simulink model "MPSK_frame_based"  (R2017b)
settings: Solver=FixedStepAuto  StartTime=0.0  StopTime=1  FixedStep=1/sampleRate  RelTol=1e-3
values from neighbouring files (symbols this model uses):
  detectionThreshold = 0.5    [MPSK_frame_based_init.m]    (also in MPSK_sample_based_init.m)
  M = 2^K    (= 4)    [Digital_QAM.m]    (also in MPSK_constellation_decisionRegions.m = 8; MPSK_frame_based_init.m = 2; MPSK_init.m = 2; MPSK_sample_based_init.m = 2)
  phaseOffset = pi    (= 3.14159265359)    [MPSK_frame_based_init.m]    (also in MPSK_init.m = -0.785398163397; MPSK_sample_based_init.m)
  sampleRate = 100    [MPSK_frame_based_init.m]    (also in MPSK_sample_based_init.m)
undefined symbols (not defined in the file or in its folder): i
libraries: simulink_extras x3, commutil2 x3, simulink x2, commfilt2 x2, commchan3 x1, dspsigops x1, commseqgen3 x1, commsink2 x1, commrflib2 x1, commrandsrc3 x1
settings Model: Creator=john3  LastModifiedBy=croft

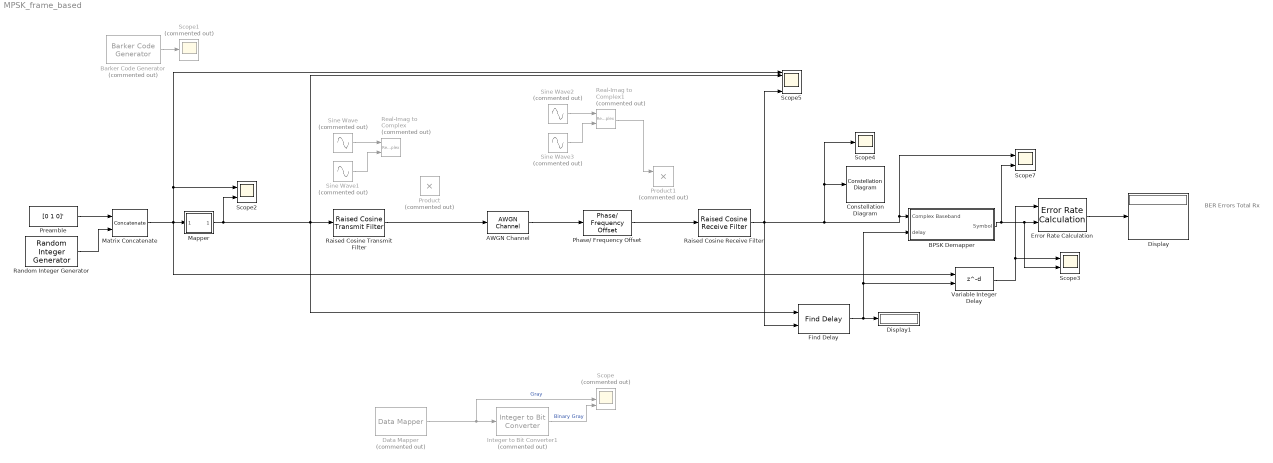
== system MPSK_frame_based ==
  note: BER
      | Errors
      | Total Rx
  AWGN Channel : commchan3/AWGN Channel  InputProcessing=Columns as channels (frame based)  seed=67  noiseMode="Signal to noise ratio  (SNR)"  EbNodB=10  EsNodB=10  SNRdB=30  bitsPerSym=K  Ps=1  Tsym=1  variance=1
  BPSK Demapper : Subsystem
  Barker Code Generator : commseqgen3/Barker Code Generator  Commented=on  Length=7  LengthSimulink=7  SampleTime=1  SamplesPerFrame=1  OutputDataType=double  SimulateUsing=Interpreted execution
      settings: SourceProductName=Communications System Toolbox  SourceProductBaseCode=CM
  Constellation Diagram : ConstellationDiagram
  Data Mapper : commutil2/Data Mapper  Commented=on  MapMode=Binary to Gray  M=M  MapVec=[0 1 3 2 7 6 4 5]
      settings: SourceProductName=Communications System Toolbox  SourceProductBaseCode=CM
  Display : Display
  Display1 : Display
  Error Rate Calculation : commsink2/Error Rate Calculation  N=0  st_delay=0  cp_mode=Entire frame  subframe=[]  PMode=Port  WsName=ErrorVec  RsMode2=off  stop=off  numErr=100  maxBits=1e6
  Find Delay : commutil2/Find Delay  corrLength=100  chgSigOP=off  stopUpdate=off  numConstDelay=3
      settings: SourceProductName=Communications System Toolbox  SourceProductBaseCode=CM
  Integer to Bit Converter1 : commutil2/Integer to Bit Converter  Commented=on  nbits=K  signedInputValues=Unsigned  bitOrder=MSB first  outDtype=Inherit via internal rule
  Mapper : Subsystem
  Matrix Concatenate : Concatenate  Mode=Multidimensional array
  Phase/ Frequency Offset : commrflib2/Phase// Frequency Offset  phaseOffset=phaseOffset*180/pi  freqPort=off  freqOffset=0
      settings: SourceProductName=Communications System Toolbox
  Preamble : Constant  Value=[0 1 0]'  SampleTime=1
  Product : Product  Commented=on
  Product1 : Product  Commented=on
  Raised Cosine Receive Filter : commfilt2/Raised Cosine Receive Filter  filtType=Square root  R=1  filtSpan=4  N=10  downFactor=10  downOffset=0  filterGain=1  InputProcessing=Columns as channels (frame based)  RateOptions=Enforce single-rate processing  framing=Mute  checkCoeff=off  variableName=rcRxFilt  currentFiltSpan=4  D=(4)/2  inputOffset=0  sampMode=Mute  saveAsFlag=0  rateMode=Downsampling  checkGain=Normalized  launchFVT=on  roundingMode=Floor  overflowMode=off  coeffDataTypeStr=Inherit: Same word length as input  coeffMin=[]  coeffMax=[]  coeffLastDataTypeStr=Inherit: Same word length as input  accumDataTypeStr=Inherit: Same as product output  accumLastDataTypeStr=Inherit: Same as product output  outputDataTypeStr=Inherit: Same as accumulator  outputMin=[]  outputMax=[]  outputLastDataTypeStr=Inherit: Same as accumulator
  Raised Cosine Transmit Filter : commfilt2/Raised Cosine Transmit Filter  filtType=Square root  R=1  filtSpan=4  N=10  filterGain=1  InputProcessing=Columns as channels (frame based)  RateOptions=Enforce single-rate processing  framing=Mute  checkCoeff=off  variableName=rcTxFilt  checkGain=Normalized  sampMode=Mute  saveAsFlag=0  currentFiltSpan=4  D=(4)/2  launchFVT=on  roundingMode=Floor  overflowMode=off  coeffDataTypeStr=Inherit: Same word length as input  coeffMin=[]  coeffMax=[]  coeffLastDataTypeStr=Inherit: Same word length as input  outputDataTypeStr=Inherit: Same as accumulator  outputMin=[]  outputMax=[]  outputLastDataTypeStr=Inherit: Same as accumulator
  Random Integer Generator : commrandsrc3/Random Integer Generator  SetSize=M  SeedSource=Auto  Seed=0  SampleTime=sampleRate  SamplesPerFrame=97  OutputDataType=double  SimulateUsing=Interpreted execution
  Real-Imag to Complex : RealImagToComplex  Commented=on
  Real-Imag to Complex1 : RealImagToComplex  Commented=on
  Scope : Scope  Commented=on  NumInputPorts=3
  Scope1 : Scope  Commented=on
  Scope2 : Scope  NumInputPorts=2
  Scope3 : Scope  NumInputPorts=2
  Scope4 : Scope
  Scope5 : Scope  NumInputPorts=7
  Scope7 : Scope  NumInputPorts=2
  Sine Wave : Sin  Commented=on  Phase=pi/2  SampleTime=0
  Sine Wave1 : Sin  Commented=on  SampleTime=0
  Sine Wave2 : Sin  Commented=on  Phase=pi/2  SampleTime=0
  Sine Wave3 : Sin  Commented=on  SampleTime=0
  Variable Integer Delay : Delay  DelayLengthSource=Input port  InputProcessing=Columns as channels (frame based)
      settings: InputPortMap=u0,p1
  wires:
  Data Mapper/1 -> Scope/2, Integer to Bit Converter1/1  "Gray"
  Integer to Bit Converter1/1 -> Scope/3  "Binary Gray"
  Raised Cosine Receive Filter/1 -> Scope5/7, Find Delay/2, Scope4/1, Constellation Diagram/1, Scope7/1, BPSK Demapper/1(Complex Baseband)
  BPSK Demapper/1(Symbol) -> Scope7/2, Scope3/2, Error Rate Calculation/2
  Error Rate Calculation/1 -> Display/1
  Barker Code Generator/1 -> Scope1/1
  Preamble/1 -> Matrix Concatenate/1
  Random Integer Generator/1 -> Matrix Concatenate/2
  Matrix Concatenate/1 -> Variable Integer Delay/1, Scope5/1, Scope2/1, Mapper/1(In1)
  Mapper/1(Out1) -> Scope5/2, Find Delay/1, Raised Cosine Transmit Filter/1, Scope2/2
  Find Delay/1 -> BPSK Demapper/2(delay), Variable Integer Delay/2, Display1/1
  Variable Integer Delay/1 -> Scope3/1, Error Rate Calculation/1
  AWGN Channel/1 -> Phase/ Frequency Offset/1
  Sine Wave/1 -> Real-Imag to Complex/1
  Sine Wave1/1 -> Real-Imag to Complex/2
  Raised Cosine Transmit Filter/1 -> AWGN Channel/1
  Sine Wave3/1 -> Real-Imag to Complex1/2
  Sine Wave2/1 -> Real-Imag to Complex1/1
  Phase/ Frequency Offset/1 -> Raised Cosine Receive Filter/1
  Real-Imag to Complex1/1 -> Product1/1

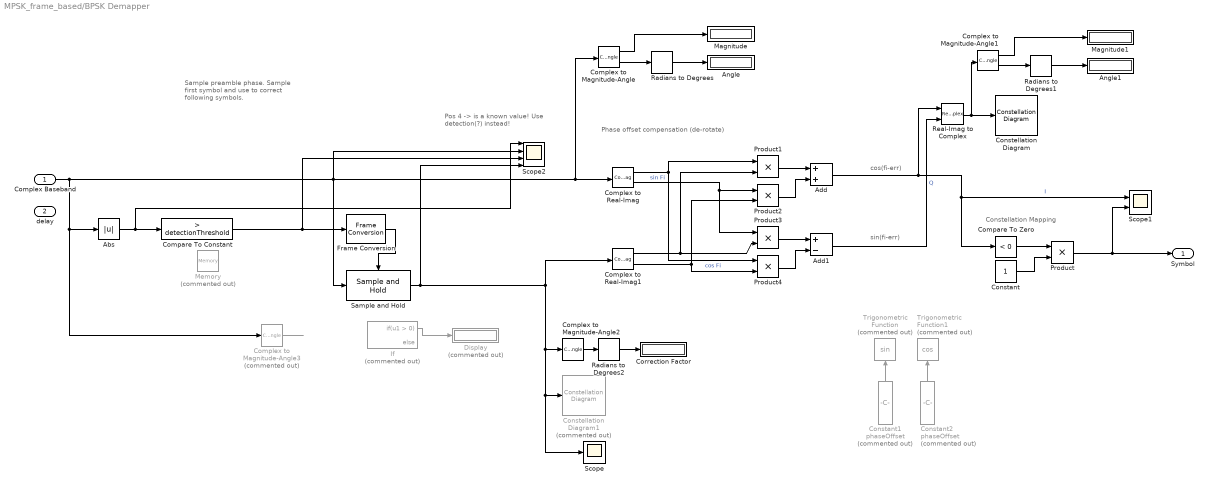
== system MPSK_frame_based/BPSK Demapper ==
  note: Pos 4 ->
      | is a known value!
      | Use detection(?)
      | instead!
  note: cos(fi-err)
  note: Sample preamble phase.
      | Sample first symbol and
      | use to correct following
      | symbols.
  note: Phase offset compensation (de-rotate)
  note: Constellation Mapping
  note: sin(fi-err)
  Complex Baseband : Inport
  delay : Inport  Port=2
  Abs : Abs
  Add : Sum
  Add1 : Sum  Inputs=+-
  Angle : Display
  Angle1 : Display
  Compare To Constant : simulink/Logic and Bit Operations/Compare To Constant  relop=>  const=detectionThreshold  OutDataTypeStr=boolean
  Compare To Zero : simulink/Logic and Bit Operations/Compare To Zero  relop=<  OutDataTypeStr=boolean
  Complex to Magnitude-Angle : ComplexToMagnitudeAngle
  Complex to Magnitude-Angle1 : ComplexToMagnitudeAngle
  Complex to Magnitude-Angle2 : ComplexToMagnitudeAngle  Output=Angle
  Complex to Magnitude-Angle3 : ComplexToMagnitudeAngle  Commented=on  Output=Angle
  Complex to Real-Imag : ComplexToRealImag
  Complex to Real-Imag1 : ComplexToRealImag
  Constant : Constant
  Constant1 : Constant  Commented=on  Value=phaseOffset
  Constant2 : Constant  Commented=on  Value=phaseOffset
  Constellation Diagram : ConstellationDiagram
  Constellation Diagram1 : ConstellationDiagram  Commented=on
  Correction Factor : Display
  Display : Display  Commented=on
  Frame Conversion : FrameConversion  InheritSamplingMode=off  OutFrame=Sample-based
  If : If  Commented=on
  Magnitude : Display
  Magnitude1 : Display
  Memory : Memory  Commented=on
  Product{,1..4} (5 alike) : Product
  Radians to Degrees : simulink_extras/Transformations/Radians to Degrees
  Radians to Degrees1 : simulink_extras/Transformations/Radians to Degrees
  Radians to Degrees2 : simulink_extras/Transformations/Radians to Degrees
  Real-Imag to Complex : RealImagToComplex
  Sample and Hold : dspsigops/Sample and Hold  trig=Rising edge  initCond=0  latchinput=on
  Scope : Scope
  Scope1 : Scope  NumInputPorts=2
  Scope2 : Scope  NumInputPorts=4
  Trigonometric Function : Trigonometry  Commented=on
  Trigonometric Function1 : Trigonometry  Commented=on  Operator=cos
  Symbol : Outport
  wires:
  Compare To Zero/1 -> Product/1
  Complex Baseband/1 -> Sample and Hold/1, Scope2/2, Complex to Magnitude-Angle/1, Complex to Real-Imag/1, Complex to Magnitude-Angle3/1, Abs/1
  Constant/1 -> Product/2
  Constant1/1 -> Trigonometric Function/1
  Constant2/1 -> Trigonometric Function1/1
  Real-Imag to Complex/1 -> Complex to Magnitude-Angle1/1, Constellation Diagram/1
  Product1/1 -> Add/1
  Product2/1 -> Add/2
  Product3/1 -> Add1/1
  Product4/1 -> Add1/2
  Add/1 -> Scope1/1, Compare To Zero/1, Real-Imag to Complex/1  "I"
  Add1/1 -> Real-Imag to Complex/2  "Q"
  Product/1 -> Scope1/2, Symbol/1
  Sample and Hold/1 -> Scope2/4, Scope/1, Constellation Diagram1/1, Complex to Magnitude-Angle2/1, Complex to Real-Imag1/1
  Complex to Magnitude-Angle/1 -> Magnitude/1
  Complex to Magnitude-Angle/2 -> Radians to Degrees/1
  Radians to Degrees/1 -> Angle/1
  Radians to Degrees1/1 -> Angle1/1
  Complex to Magnitude-Angle1/2 -> Radians to Degrees1/1
  Complex to Magnitude-Angle1/1 -> Magnitude1/1
  Complex to Magnitude-Angle2/1 -> Radians to Degrees2/1
  Radians to Degrees2/1 -> Correction Factor/1
  Complex to Real-Imag/1 -> Product4/1, Product1/1  "cos Fi"
  Complex to Real-Imag1/1 -> Product3/2, Product1/2
  Complex to Real-Imag/2 -> Product3/1, Product2/1  "sin Fi"
  Complex to Real-Imag1/2 -> Product4/2, Product2/2
  If/1 -> Display/1
  Complex to Magnitude-Angle3/1 -> ?
  ? -> If/1
  Abs/1 -> Scope2/1, Compare To Constant/1
  Compare To Constant/1 -> Scope2/3, Frame Conversion/1
  Frame Conversion/1 -> Sample and Hold/Trigger

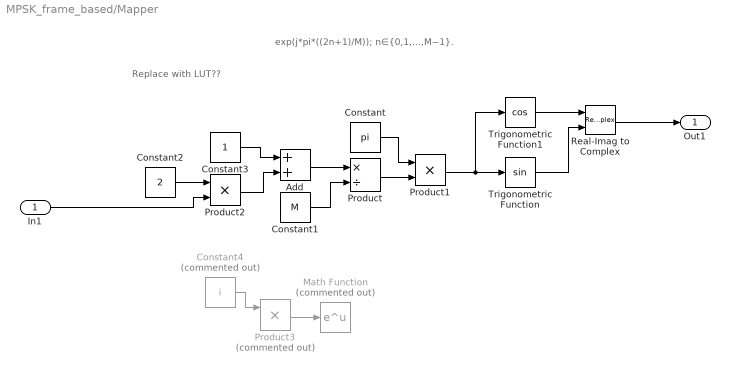
== system MPSK_frame_based/Mapper ==
  note: Replace with LUT??
  note: exp(j*pi*((2n+1)/M)); n∈{0,1,…,M−1}.
  In1 : Inport
  Add : Sum
  Constant : Constant  Value=pi
  Constant1 : Constant  Value=M
  Constant2 : Constant  Value=2
  Constant3 : Constant
  Constant4 : Constant  Commented=on  Value=i
  Math Function : Math  Commented=on  SaturateOnIntegerOverflow=on
  Product : Product  Inputs=*/
  Product1 : Product
  Product2 : Product
  Product3 : Product  Commented=on
  Real-Imag to Complex : RealImagToComplex
  Trigonometric Function : Trigonometry  ApproximationMethod=CORDIC
  Trigonometric Function1 : Trigonometry  Operator=cos  ApproximationMethod=CORDIC
  Out1 : Outport
  wires:
  Real-Imag to Complex/1 -> Out1/1
  Constant2/1 -> Product2/1
  In1/1 -> Product2/2
  Product1/1 -> Trigonometric Function1/1, Trigonometric Function/1
  Trigonometric Function1/1 -> Real-Imag to Complex/1
  Add/1 -> Product/1
  Product/1 -> Product1/2
  Constant3/1 -> Add/1
  Constant1/1 -> Product/2
  Trigonometric Function/1 -> Real-Imag to Complex/2
  Product2/1 -> Add/2
  Constant/1 -> Product1/1
  Constant4/1 -> Product3/1
  Product3/1 -> Math Function/1
